simulink model "mpcACCsystem"  (R2023a)
settings: Solver=FixedStepAuto  StartTime=0.0  StopTime=T  RelTol=1e-3
values from neighbouring files (symbols this model uses):
  t_gap = 1.4    [AdaptiveCruiseControlExample.m]
  Ts = 0.1    [AdaptiveCruiseControlExample.m]
  v0_ego = 20    [AdaptiveCruiseControlExample.m]
  v0_lead = 25    [AdaptiveCruiseControlExample.m]
  v_set = 30    [AdaptiveCruiseControlExample.m]
  x0_ego = 10    [AdaptiveCruiseControlExample.m]
  x0_lead = 50    [AdaptiveCruiseControlExample.m]
undefined symbols (not defined in the file or in its folder): max_ac, min_ac, verr_gain, vx_gain, xerr_gain
settings Model: Creator=The MathWorks, Inc.  LastModifiedBy=Leo
settings SolverCC: AlgebraicLoopSolver=TrustRegion
settings DataIOCC: ReturnWorkspaceOutputs=off
settings DebuggingCC: UnconnectedInputMsg=warning  UnconnectedOutputMsg=warning  UnconnectedLineMsg=warning  ArithmeticOperatorsInVariantConditions=warning
settings ModelReferenceCC: EnableRefExpFcnMdlSchedulingChecks=on
settings SFSimCC: SimUseLocalCustomCode=off  CustomCodeUndefinedFunction=UseInterfaceOnly
settings RTWCC: RTWUseLocalCustomCode=off
settings CodeAppCC: StateflowObjectComments=on

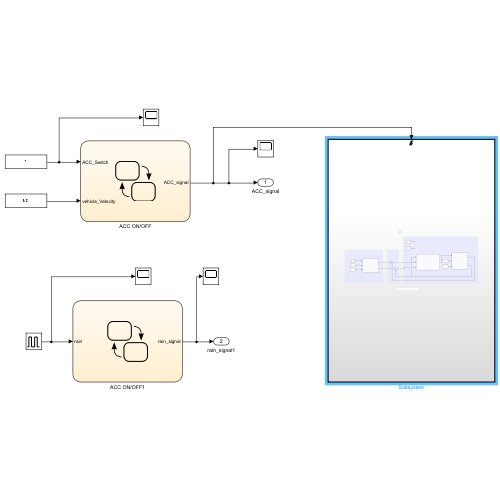
[thumbnail: Simulink's stored preview of the top-level diagram]
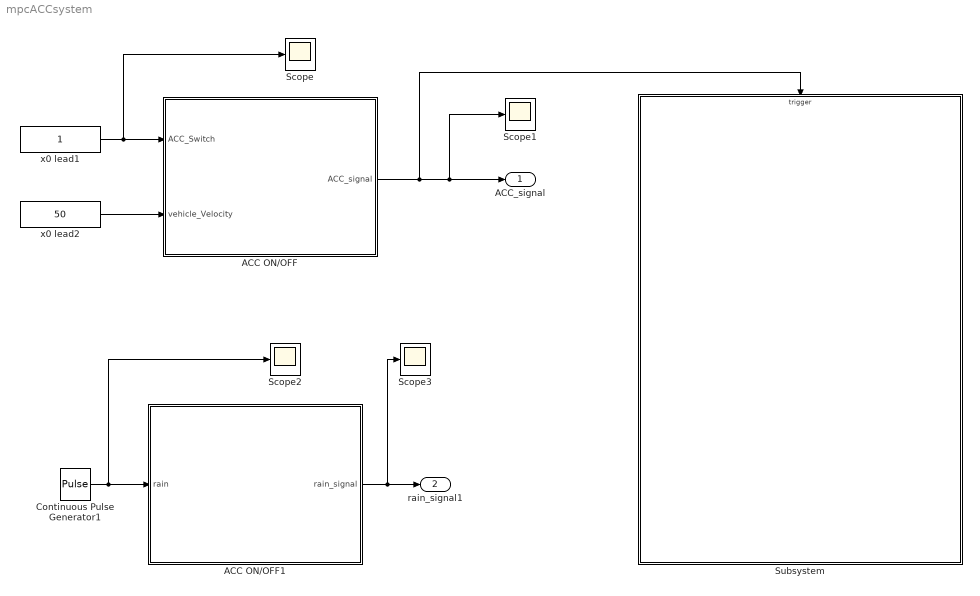
== system mpcACCsystem ==
  ACC ON/OFF : Stateflow chart  TreatAsAtomicUnit=on
  ACC ON/OFF1 : Stateflow chart  TreatAsAtomicUnit=on
  Continuous Pulse Generator1 : DiscretePulseGenerator  PulseType=Time based  Period=20  PulseWidth=50
  Scope{,1..3} (4 alike) : Scope
  Subsystem : Subsystem
  x0 lead1 : Constant  SampleTime=Ts
  x0 lead2 : Constant  Value=50  SampleTime=Ts
  ACC_signal : Outport  VectorParamsAs1DForOutWhenUnconnected=off
  rain_signal1 : Outport  Port=2  VectorParamsAs1DForOutWhenUnconnected=off
  wires:
  x0 lead1/1 -> Scope/1, ACC ON/OFF/1(ACC_Switch)
  x0 lead2/1 -> ACC ON/OFF/2(vehicle_Velocity)
  ACC ON/OFF/1(ACC_signal) -> Subsystem/Trigger, ACC_signal/1, Scope1/1
  Continuous Pulse Generator1/1 -> ACC ON/OFF1/1(rain), Scope2/1
  ACC ON/OFF1/1(rain_signal) -> Scope3/1, rain_signal1/1

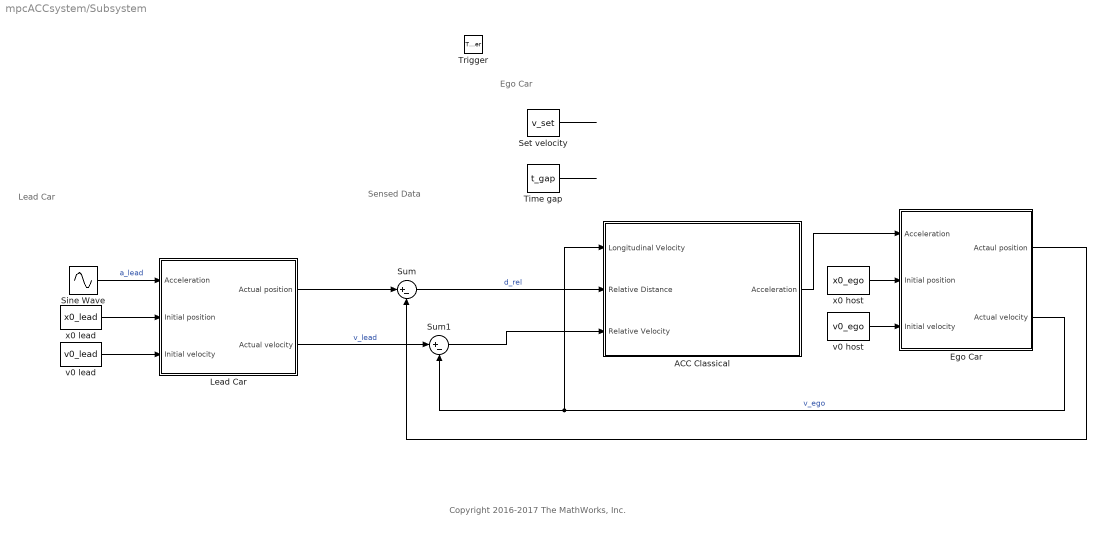
== system mpcACCsystem/Subsystem ==
  note: Sensed Data
  note: Lead Car
  note: Ego Car
  note: Copyright 2016-2017 The MathWorks, Inc.
  Trigger : TriggerPort  VariantControl=(inherit)  PortDimensions=1
  ACC Classical : Subsystem  TreatAsAtomicUnit=on  VariantControl=controller_type == 1
      settings: RTWFileNameOpts=Use function name
  Ego Car : Subsystem
  Lead Car : Subsystem
  Set velocity : Constant  Value=v_set  SampleTime=Ts
  Sine Wave : Sin  Amplitude=0.6  Frequency=0.2  SampleTime=Ts
  Sum : Sum  Inputs=|+-
  Sum1 : Sum  Inputs=|+-
  Time gap : Constant  Value=t_gap  SampleTime=Ts
  v0 host : Constant  Value=v0_ego  SampleTime=Ts
  v0 lead : Constant  Value=v0_lead  SampleTime=Ts
  x0 host : Constant  Value=x0_ego  SampleTime=Ts
  x0 lead : Constant  Value=x0_lead  SampleTime=Ts
  wires:
  Sum/1 -> ACC Classical/2(Relative Distance)  "d_rel"
  v0 lead/1 -> Lead Car/3(Initial velocity)
  x0 host/1 -> Ego Car/2(Initial position)
  Set velocity/1 -> ?
  Sine Wave/1 -> Lead Car/1(Acceleration)  "a_lead"
  Ego Car/2(Actual velocity) -> ACC Classical/1(Longitudinal Velocity), Sum1/2  "v_ego"
  Sum1/1 -> ACC Classical/3(Relative Velocity)
  Ego Car/1(Actaul position) -> Sum/2
  v0 host/1 -> Ego Car/3(Initial velocity)
  Time gap/1 -> ?
  Lead Car/2(Actual velocity) -> Sum1/1  "v_lead"
  x0 lead/1 -> Lead Car/2(Initial position)
  Lead Car/1(Actual position) -> Sum/1
  ACC Classical/1(Acceleration) -> Ego Car/1(Acceleration)

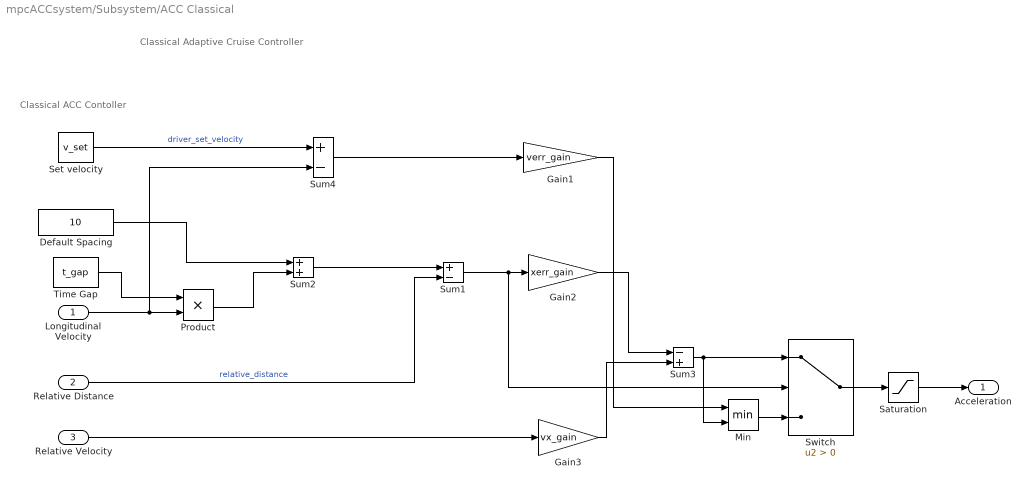
== system mpcACCsystem/Subsystem/ACC Classical ==
  note: Classical ACC Contoller
  note: Classical Adaptive Cruise Controller
  Longitudinal Velocity : Inport
  Relative Distance : Inport  Port=2
  Relative Velocity : Inport  Port=3
  Default Spacing : Constant  Value=10  SampleTime=Ts
  Gain1 : Gain  Gain=verr_gain
  Gain2 : Gain  Gain=xerr_gain
  Gain3 : Gain  Gain=vx_gain
  Min : MinMax  Inputs=2
  Product : Product
  Saturation : Saturate  UpperLimit=max_ac  LowerLimit=min_ac
  Set velocity : Constant  Value=v_set  SampleTime=Ts
  Sum1 : Sum  Inputs=+-
  Sum2 : Sum
  Sum3 : Sum  Inputs=-+
  Sum4 : Sum  Inputs=+-
  Switch : Switch  Criteria=u2 > Threshold  SaturateOnIntegerOverflow=off  InputSameDT=off
  Time Gap : Constant  Value=t_gap  SampleTime=Ts
  Acceleration : Outport  VectorParamsAs1DForOutWhenUnconnected=off
  wires:
  Longitudinal Velocity/1 -> Product/2, Sum4/2
  Default Spacing/1 -> Sum2/1
  Gain2/1 -> Sum3/1
  Sum4/1 -> Gain1/1
  Min/1 -> Switch/3
  Gain3/1 -> Sum3/2
  Switch/1 -> Saturation/1
  Relative Velocity/1 -> Gain3/1
  Time Gap/1 -> Product/1
  Saturation/1 -> Acceleration/1
  Product/1 -> Sum2/2
  Set velocity/1 -> Sum4/1  "driver_set_velocity"
  Sum3/1 -> Min/2, Switch/1
  Sum1/1 -> Switch/2, Gain2/1
  Gain1/1 -> Min/1
  Relative Distance/1 -> Sum1/2  "relative_distance"
  Sum2/1 -> Sum1/1

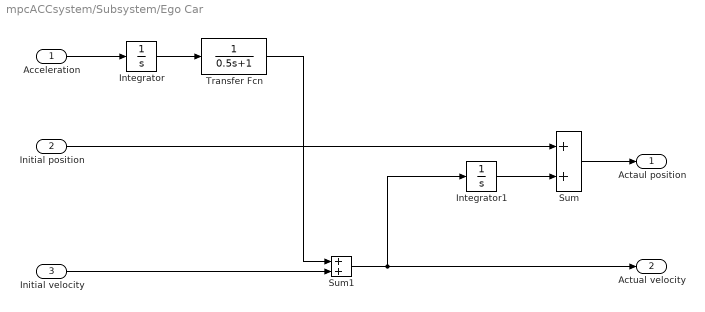
== system mpcACCsystem/Subsystem/Ego Car ==
  Acceleration : Inport
  Initial position : Inport  Port=2
  Initial velocity : Inport  Port=3
  Integrator : Integrator
  Integrator1 : Integrator
  Sum : Sum
  Sum1 : Sum
  Transfer Fcn : TransferFcn  Denominator=[0.5 1]
  Actaul position : Outport  VectorParamsAs1DForOutWhenUnconnected=off
  Actual velocity : Outport  Port=2  VectorParamsAs1DForOutWhenUnconnected=off
  wires:
  Sum1/1 -> Integrator1/1, Actual velocity/1
  Initial velocity/1 -> Sum1/2
  Sum/1 -> Actaul position/1
  Transfer Fcn/1 -> Sum1/1
  Integrator/1 -> Transfer Fcn/1
  Acceleration/1 -> Integrator/1
  Initial position/1 -> Sum/1
  Integrator1/1 -> Sum/2

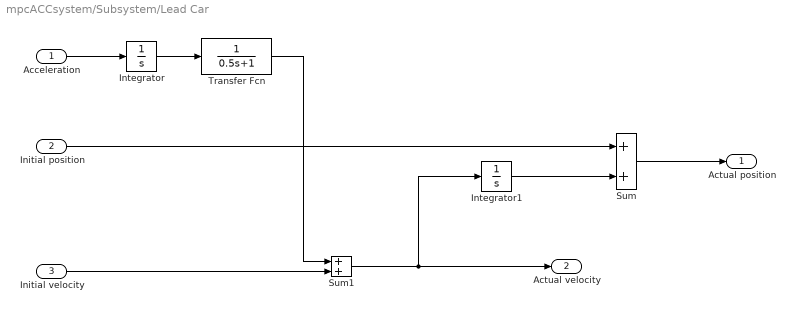
== system mpcACCsystem/Subsystem/Lead Car ==
  Acceleration : Inport
  Initial position : Inport  Port=2
  Initial velocity : Inport  Port=3
  Integrator : Integrator
  Integrator1 : Integrator
  Sum : Sum
  Sum1 : Sum
  Transfer Fcn : TransferFcn  Denominator=[0.5 1]
  Actual position : Outport  VectorParamsAs1DForOutWhenUnconnected=off
  Actual velocity : Outport  Port=2  VectorParamsAs1DForOutWhenUnconnected=off
  wires:
  Transfer Fcn/1 -> Sum1/1
  Initial velocity/1 -> Sum1/2
  Sum/1 -> Actual position/1
  Integrator/1 -> Transfer Fcn/1
  Sum1/1 -> Integrator1/1, Actual velocity/1
  Acceleration/1 -> Integrator/1
  Initial position/1 -> Sum/1
  Integrator1/1 -> Sum/2

== stateflow chart mpcACCsystem/ACC ON//OFF1 ==
  state no_rain
    entry:
    rain_signal = 0;
  state rain
    entry:
    rain_signal = 1;
  (default) -> no_rain
  no_rain -> rain : [rain == 1]
  rain -> no_rain : [rain == 0]
  data: rain input; rain_signal output

== stateflow chart mpcACCsystem/ACC ON//OFF ==
  state ACC_OFF
    entry:
    ACC_signal = 0;
  state ACC_ON
    entry:
    ACC_signal = 1;
  (default) -> ACC_OFF
  ACC_OFF -> ACC_ON : [ACC_Switch == 1 && vehicle_Velocity >= 40]
  ACC_ON -> ACC_OFF : [ACC_Switch == 0 || vehicle_Velocity >= 120]
  data: ACC_signal output; ACC_Switch input; vehicle_Velocity input
